simulink model "UdpPacketsSplit"  (Simulink 7.7)
settings: Solver=FixedStepDiscrete  StartTime=0.0  StopTime=10.0  FixedStep=0.01  RelTol=1e-3
libraries: UAVdesign_net x5
settings Model: Creator=Emanuel  LastModifiedBy=Emanuel

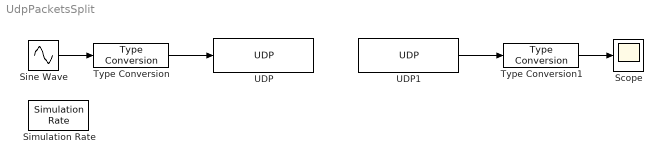
== system UdpPacketsSplit ==
  Scope : Scope
      settings: YMin=-2  YMax=2
  Simulation Rate : UAVdesign_net/Hardware/Simulation Rate  SimSampleTime=1/100
  Sine Wave : Sin  Frequency=2*pi  SampleTime=0
  Type Conversion : UAVdesign_net/Hardware/Type Conversion  indim=1  intype=double  outdim=8  outtype=uint8  signextend=off
  Type Conversion1 : UAVdesign_net/Hardware/Type Conversion  indim=8  intype=uint8  outdim=1  outtype=double  signextend=off
  UDP : UAVdesign_net/Hardware/UDP  host='localhost'  remote_port=60500  local_port=60400  timeout=0  tx_enable=on  rx_enable=off  receive=8  num_packets_overrun=off  num_packets_received=off  handshake=off  st=-1
  UDP1 : UAVdesign_net/Hardware/UDP  host='localhost'  remote_port=60200  local_port=60500  timeout=0  tx_enable=off  rx_enable=on  receive=8  num_packets_overrun=off  num_packets_received=off  handshake=off  st=-1
  wires:
  Sine Wave/1 -> Type Conversion/1
  Type Conversion/1 -> UDP/1
  Type Conversion1/1 -> Scope/1
  UDP1/1 -> Type Conversion1/1
